simulink model "ComparadorModelo_continuo_cascada"  (Simulink 8.0)
settings: Solver=ode45  StartTime=0.0  StopTime=exp(end,1)  FixedStep=0.06  MaxStep=0.06  RelTol=1e-4
undefined symbols (not defined in the file or in its folder): DiscIntNeverNeededParam, Ts
libraries: slident x2
settings Model: Creator=sergarro  LastModifiedBy=Carlos
settings DataIOCC: SignalLoggingSaveFormat=ModelDataLogs
settings DebuggingCC: FcnCallInpInsideContextMsg=UseLocalSettings  StrictBusMsg=Warning
settings GRTTargetCC: CombineOutputUpdateFcns=off  GRTInterface=on

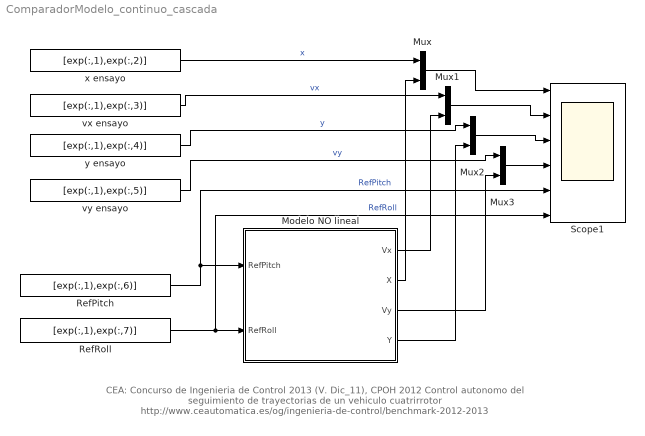
== system ComparadorModelo_continuo_cascada ==
  note: CEA: Concurso de Ingenieria de Control 2013 (V. Dic_11), CPOH 2012
      | Control autonomo del seguimiento de trayectorias de un vehiculo cuatrirrotor
      | http://www.ceautomatica.es/og/ingenieria-de-control/benchmark-2012-2013
  " Modelo NO lineal" : Subsystem
  Mux{,1..3} (4 alike) : Mux  Inputs=2
  RefPitch : FromWorkspace  VariableName=[exp(:,1),exp(:,6)]  SampleTime=0.06
  RefRoll : FromWorkspace  VariableName=[exp(:,1),exp(:,7)]  SampleTime=0.06
  Scope1 : Scope  NumInputPorts=6
      settings: TimeRange=800  YMin=-40~-5~-20~-5~-1~-1  YMax=20~5~40~5~1~1  SaveName=ResultExp  MaxDataPoints=15000  SampleInput=on  SampleTime=0.06
  vx ensayo : FromWorkspace  VariableName=[exp(:,1),exp(:,3)]  SampleTime=0.06
  vy ensayo : FromWorkspace  VariableName=[exp(:,1),exp(:,5)]  SampleTime=0.06
  x ensayo : FromWorkspace  VariableName=[exp(:,1),exp(:,2)]  SampleTime=0.06
  y ensayo : FromWorkspace  VariableName=[exp(:,1),exp(:,4)]  SampleTime=0.06
  wires:
  RefRoll/1 -> Scope1/6, " Modelo NO lineal"/2(RefRoll)  "RefRoll"
  RefPitch/1 -> " Modelo NO lineal"/1(RefPitch), Scope1/5  "RefPitch"
  Mux/1 -> Scope1/1
  x ensayo/1 -> Mux/1  "x"
  " Modelo NO lineal"/2(X) -> Mux/2
  vx ensayo/1 -> Mux1/1  "vx"
  " Modelo NO lineal"/1(Vx) -> Mux1/2
  Mux1/1 -> Scope1/2
  y ensayo/1 -> Mux2/1  "y"
  " Modelo NO lineal"/4(Y) -> Mux2/2
  Mux2/1 -> Scope1/3
  Mux3/1 -> Scope1/4
  " Modelo NO lineal"/3(Vy) -> Mux3/2
  vy ensayo/1 -> Mux3/1  "vy"

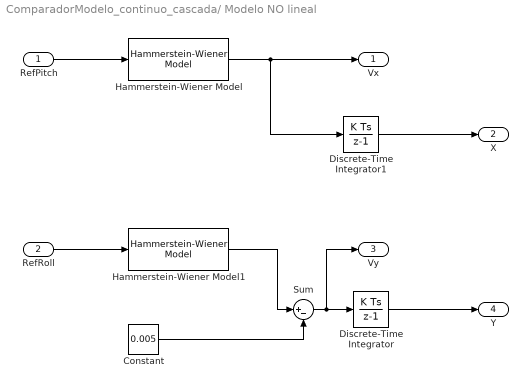
== system ComparadorModelo_continuo_cascada/ Modelo NO lineal ==
  RefPitch : Inport  PortDimensions=1  SampleTime=0.06
  RefRoll : Inport  Port=2  PortDimensions=1  SampleTime=0.06
  Constant : Constant  Value=0.005
  Discrete-Time Integrator : DiscreteIntegrator  gainval=1  InitialCondition=-1  SampleTime=Ts  ICPrevOutput=DiscIntNeverNeededParam  ICPrevScaledInput=DiscIntNeverNeededParam
  Discrete-Time Integrator1 : DiscreteIntegrator  gainval=1  InitialCondition=0.5  SampleTime=Ts  ICPrevOutput=DiscIntNeverNeededParam  ICPrevScaledInput=DiscIntNeverNeededParam
  Hammerstein-Wiener Model : slident/Hammerstein-Wiener Model  sys=vx123_nlhw113_pic2  IC=Zero  X0i=0
  Hammerstein-Wiener Model1 : slident/Hammerstein-Wiener Model  sys=vy123_nlhw111  IC=Zero  X0i=0
  Sum : Sum  Inputs=|+-
  Vx : Outport
  X : Outport  Port=2
  Vy : Outport  Port=3
  Y : Outport  Port=4
  wires:
  Hammerstein-Wiener Model1/1 -> Sum/1
  Hammerstein-Wiener Model/1 -> Discrete-Time Integrator1/1, Vx/1
  RefRoll/1 -> Hammerstein-Wiener Model1/1
  RefPitch/1 -> Hammerstein-Wiener Model/1
  Discrete-Time Integrator/1 -> Y/1
  Discrete-Time Integrator1/1 -> X/1
  Constant/1 -> Sum/2
  Sum/1 -> Vy/1, Discrete-Time Integrator/1
